simulink model "distortion3"  (R2019b)
settings: Solver=VariableStepAuto  StartTime=0.0  StopTime=inf  RelTol=1e-3
undefined symbols (not defined in the file): fdesignblkfcn, gcbh
libraries: rfmathmodels1 x2, commrfcorlib x1, dspsigops x1
settings Model: PacingRate=0.089000  Creator=Dominik  LastModifiedBy=касенов

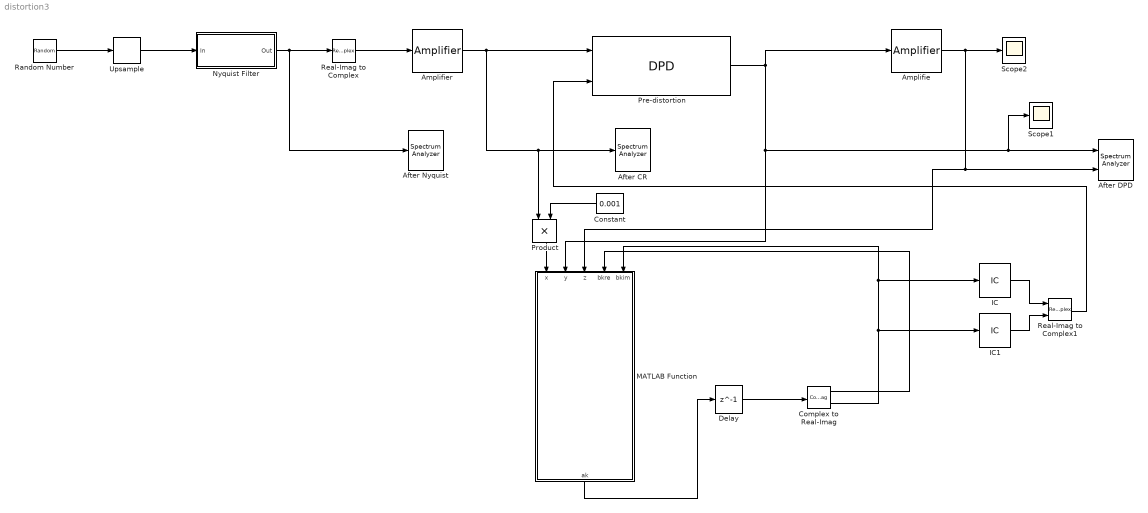
== system distortion3 ==
  After CR : SpectrumAnalyzer
  After DPD : SpectrumAnalyzer  NumInputPorts=2
  After Nyquist : SpectrumAnalyzer
  Amplifie : rfmathmodels1/Amplifier  model_select=Rapp model  linGaindB=0  GindB=0  iip3=30  am2pm=10  PwrAMPMStart=10  PwrAMPMEnd=inf  amam=[2.1587 1.1517]  ampm=[4.0033 9.1040]  x=[8.1081 1.5413 6.5202 -0.0718]  y=[4.6645 2.0965 10.88 -0.003]  p=0.5  GoutdB=0  vsat=1  method_select=Noise factor  ntemp=290  nfigure=3.01  nfactor=2  seed=67987
      settings: SourceProductName=RF Blockset  SourceProductBaseCode=RB
  Amplifier : rfmathmodels1/Amplifier  model_select=Rapp model  linGaindB=0  GindB=0  iip3=30  am2pm=10  PwrAMPMStart=10  PwrAMPMEnd=inf  amam=[2.1587 1.1517]  ampm=[4.0033 9.1040]  x=[8.1081 1.5413 6.5202 -0.0718]  y=[4.6645 2.0965 10.88 -0.003]  p=2  GoutdB=0  vsat=1  method_select=Noise factor  ntemp=290  nfigure=3.01  nfactor=2  seed=67987
      settings: SourceProductName=RF Blockset  SourceProductBaseCode=RB
  Complex to Real-Imag : ComplexToRealImag
  Constant : Constant  Value=0.001
  Delay : Delay  DelayLength=1  InitialCondition=0  UseCircularBuffer=on
  IC : InitialCondition
  IC1 : InitialCondition
  MATLAB Function : MATLAB Function  TreatAsAtomicUnit=on
  Nyquist Filter : Subsystem  DialogController=fdesignblkfcn  InitFcn=fdesignblkfcn(gcbh, {'InitFcn'});  mask(Nyquist Filter){}
      mask help: Design a Nyquist filter
      settings: CopyFcn=fdesignblkfcn(gcbh, {'CopyFcn'});
      mask Help: helpview(mapfilelocation('dsp'), 'dspnyquistfilter');
      mask Display: disp('Nyquist');
  Pre-distortion : commrfcorlib/DPD  PolynomialType=Memory polynomial  CoefficientSource=Input port  Coefficients=complex([1 0 0 0 0; 0 0 0 0 0; 0 0 0 0 0])  SimulateUsing=Code generation
      settings: SourceProductName=Communications Toolbox  SourceProductBaseCode=CM
  Product : Product
  Random Number : RandomNumber  SampleTime=0.001
  Real-Imag to Complex : RealImagToComplex  Input=Real
  Real-Imag to Complex1 : RealImagToComplex
  Scope1 : Scope
  Scope2 : Scope
  Upsample : dspsigops/Upsample  N=8  phase=0  RateOptions=Allow multirate processing  ic=0  mode=Unused parameter value
  wires:
  Real-Imag to Complex/1 -> Amplifier/1
  Random Number/1 -> Upsample/1
  Upsample/1 -> Nyquist Filter/1(In)
  Nyquist Filter/1(Out) -> Real-Imag to Complex/1, After Nyquist/1
  Pre-distortion/1 -> Amplifie/1, MATLAB Function/2(y), Scope1/1, After DPD/1
  Amplifie/1 -> Scope2/1, MATLAB Function/3(z), After DPD/2
  Product/1 -> MATLAB Function/1(x)
  Constant/1 -> Product/2
  MATLAB Function/1(ak) -> Delay/1
  Complex to Real-Imag/1 -> MATLAB Function/4(bkre)
  Complex to Real-Imag/2 -> IC1/1, IC/1, MATLAB Function/5(bkim)
  Delay/1 -> Complex to Real-Imag/1
  Amplifier/1 -> After CR/1, Product/1, Pre-distortion/1
  IC/1 -> Real-Imag to Complex1/1
  IC1/1 -> Real-Imag to Complex1/2
  Real-Imag to Complex1/1 -> Pre-distortion/2

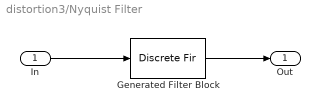
== system distortion3/Nyquist Filter ==
  In : Inport
  Generated Filter Block : DiscreteFir  Tag=BlockMethodSubSystem  Coefficients=[-1.51622726129955863e-05 0 4.17065642797130267e-05 0 -8.63974532359493069e-05 0 0.000156112339412392586 0 -0.000259152163405612895 0 0.000405340967727107018 0 -0.000606122081126900724 0 0.000874664613518894908 0 -0.00122600321576426152 0 0.00167724728876562468 0 -0.00224791534173759749 0 0.00296048017608780203 0 -0.00384125870473808143 0 0.00492186111131599595 0 -0.00624155643186620392 0 0.00785117446710228636 0 -0.00981967458384361454 0 0.0122455627766693432 0 -0.0152776505052993374 0 0.0191551639220552683 0 -0.0242917549435244136 0 0.0314715991488982369 0 -0.0423816072426853388 0 0.0614206608292716463 0 -0.104744991792953324 0 0.317854846111936151 0.5 0.317854846111936151 0 -0.104744991792953324 0 0.0614206608292716463 0 -0.0423816072426853388 0 0.0314715991488982369 0 -0.0242917549435244136 0 0.0191551639220552683 0 -0.0152776505052993374 0 0.0122455627766693432 0 -0.00981967458384361454 0 0.00785117446710228636 0 -0.00624155643186620392 0 0.00492186111131599595 0 -0.00384125870473808143 0 0.00296048017608780203 0 -0.00224791534173759749 0 0.00167724728876562468 0 -0.00122600321576426152 0 0.000874664613518894908 0 -0.000606122081126900724 0 0.000405340967727107018 0 -0.000259152163405612895 0 0.000156112339412392586 0 -8.63974532359493069e-05 0 4.17065642797130267e-05 0 -1.51622726129955863e-05]
  Out : Outport  VectorParamsAs1DForOutWhenUnconnected=off
  wires:
  In/1 -> Generated Filter Block/1
  Generated Filter Block/1 -> Out/1

== matlab function distortion3/MATLAB Function ==
  data: x input; ak output; y input; z input; bkre input; bkim input
function ak = fcn(x,y,z, bkre, bkim)

gamma = 1e-3;

x_phase = x / abs(x);
y_phase = y / abs(y);
z_phase = z / abs(z);

phase = z_phase * x_phase / y_phase;

bk = bkre + bkim;

ak = bk - gamma*(z-x)*phase;
end
% ak = bk + gamma*(z-x)*z*x/y;
